simulink model "SMA_displacementIn_spring"  (R2018a)
settings: Solver=ode15s  StartTime=0.0  StopTime=100  RelTol=1e-6  AbsTol=1e-6  EnableMultiTasking=on
InitFcn:
  | Parameter;
libraries: simulink x1
settings Model: Creator=Johannes  LastModifiedBy=Matthias
settings SolverCC: AutoScaleAbsTol=off
settings DataIOCC: LimitDataPoints=on  SaveFormat=Array  SignalLoggingSaveFormat=ModelDataLogs
settings OptimizationCC: LifeSpan=inf
settings DebuggingCC: UnderspecifiedInitializationDetection=Classic  MergeDetectMultiDrivingBlocksExec=none  SolverPrmCheckMsg=warning  MultiTaskDSMMsg=warning  MultiTaskCondExecSysMsg=none  SFUnexpectedBacktrackingDiag=warning  SFNoUnconditionalDefaultTransitionDiag=warning  SFExecutionAtInitializationDiag=none
settings HardwareCC: ProdBitPerPointer=32  ProdBitPerSizeT=32  ProdBitPerPtrDiffT=32  ProdLargestAtomicFloat=None  ProdIntDivRoundTo=Undefined  ProdEndianess=Unspecified  ProdWordSize=32  ProdHWDeviceType=32-bit Generic
settings ModelReferenceCC: PropagateSignalLabelsOutOfModel=off
settings CodeAppCC: StateflowObjectComments=on
settings GRTTargetCC: TargetLangStandard=C89/C90 (ANSI)  GeneratePreprocessorConditionals=Disable all
settings ConfigComp: CovMetricSettings=dw  CovHtmlReporting=on  CovSaveCumulativeToWorkspaceVar=on  CovSaveSingleToWorkspaceVar=on  CovExternalEMLEnable=off

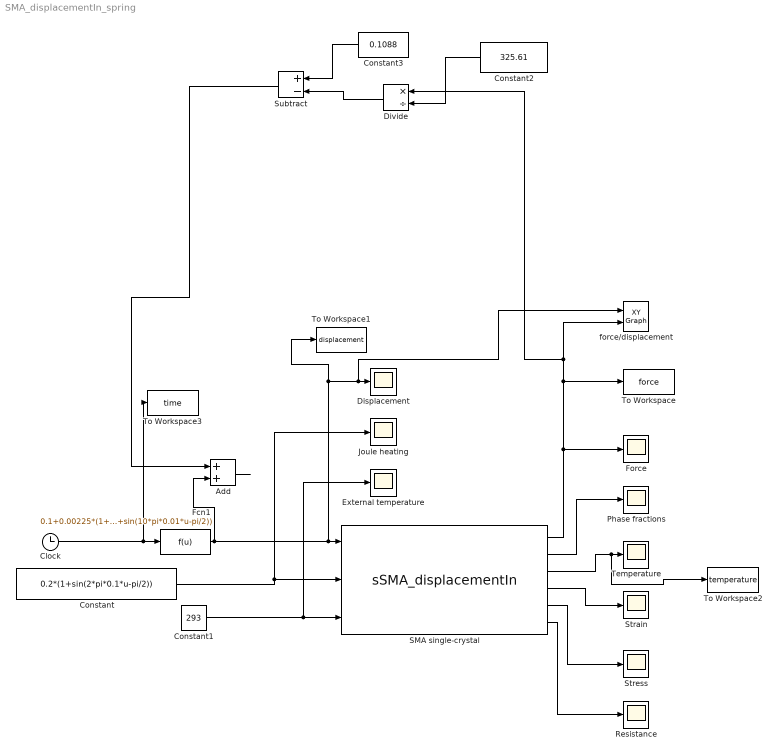
== system SMA_displacementIn_spring ==
  Add : Sum
  Clock : Clock
  Constant : Constant  Value=0.2*(1+sin(2*pi*0.1*u-pi/2))
  Constant1 : Constant  Value=293
  Constant2 : Constant  Value=325.61
  Constant3 : Constant  Value=0.1088
  Displacement : Scope
  Divide : Product  Inputs=*/
  External temperature : Scope
  Fcn1 : Fcn  Expr=0.1+0.00225*(1+sin(2*pi*0.01*u-pi/2))+0.00075*(1+sin(10*pi*0.01*u-pi/2))
  Force : Scope
  Joule heating : Scope
  Phase fractions : Scope
  Resistance : Scope
  SMA single-crystal : M-S-Function  FunctionName=sSMA_displacementIn  Parameters=params, initConds
      mask Display:
      | color('black');
      | patch(3*[-1 1 1 -1],1.1*[-1 -1 1 1],[1 1 1]);
      | patch([-1.6 -0.8],[-0.9 0.3],[0 0 0]);
      | patch([-0.8 1.2],[0.3 0.3],[0 0 0]);
      | patch([1.6 0.8],[0.9 -0.3],[0 0 0]);
      | patch([0.8 -1.2],[-0.3 -0.3],[0 0 0]);
      | disp('SMA');
      | 
      | color('blue');
      | port_label('input', 1, 'y [m]','texmode','on');
      | port_label('input', 2, 'J [W]','texmode','on');
      | port_label('input', 3, 'T_E [K]','texmode','on');
      | 
      | color('red');
      | port_label('output', 1, 'F [N]','texmode','on');
      | port_label('output', 2, 'x_+, x_-, x_A [-]','texmode','on');
      | port_label('output', 3, 'T [K]','texmode','on');
      | port_label('output', 4, '\epsilon [-]','texmode','on');
      | port_label('output', 5, '\sigma [Pa]','texmode','on');
      | port_label('output', 6, 'R [\Omega]','texmode','on');
  Strain : Scope
  Stress : Scope
  Subtract : Sum  Inputs=+-
  Temperature : Scope
  To Workspace : ToWorkspace  VariableName=force  SampleTime=-1
  To Workspace1 : ToWorkspace  VariableName=displacement  SampleTime=-1
  To Workspace2 : ToWorkspace  VariableName=temperature  SampleTime=-1
  To Workspace3 : ToWorkspace  VariableName=time  SampleTime=-1
  force/displacement : simulink/Sinks/XY Graph  xmin=0.1  xmax=0.106  ymin=0  ymax=2.5  st=-1
  wires:
  SMA single-crystal/2 -> Phase fractions/1
  SMA single-crystal/3 -> To Workspace2/1, Temperature/1
  SMA single-crystal/4 -> Strain/1
  SMA single-crystal/5 -> Stress/1
  SMA single-crystal/6 -> Resistance/1
  Clock/1 -> To Workspace3/1, Fcn1/1
  Constant/1 -> Joule heating/1, SMA single-crystal/2
  Constant1/1 -> External temperature/1, SMA single-crystal/3
  Fcn1/1 -> To Workspace1/1, force/displacement/1, Displacement/1, SMA single-crystal/1, Add/2
  Subtract/1 -> Add/1
  Divide/1 -> Subtract/2
  Constant2/1 -> Divide/2
  Constant3/1 -> Subtract/1
  SMA single-crystal/1 -> To Workspace/1, Divide/1, force/displacement/2, Force/1
  Add/1 -> ?
